simulink model "HWA1"  (R2017a)
settings: Solver=VariableStepAuto  StartTime=0.0  StopTime=10.0  RelTol=1e-3  EnableMultiTasking=on
values from neighbouring files (symbols this model uses):
  g = 9.81    [main.m]
  m = 0.4    [main.m]
settings Model: Creator=s160096  LastModifiedBy=Filip Davidovic
settings OptimizationCC: LifeSpan=inf
settings DebuggingCC: SFUnexpectedBacktrackingDiag=warning  SFNoUnconditionalDefaultTransitionDiag=warning  SFExecutionAtInitializationDiag=none
settings GRTTargetCC: TargetLangStandard=C89/C90 (ANSI)  GeneratePreprocessorConditionals=Disable all
settings ConfigComp: CovMetricSettings=dw  CovHtmlReporting=on  CovSaveCumulativeToWorkspaceVar=on  CovSaveSingleToWorkspaceVar=on  CovExternalEMLEnable=off

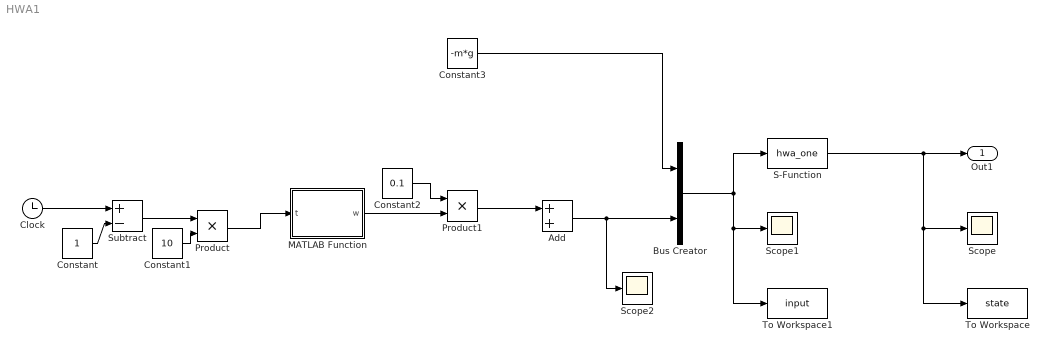
== system HWA1 ==
  Add : Sum
  Bus Creator : BusCreator  Inputs=2
  Clock : Clock
  Constant : Constant
  Constant1 : Constant  Value=10
  Constant2 : Constant  Value=0.1
  Constant3 : Constant  Value=-m*g
  MATLAB Function : MATLAB Function  TreatAsAtomicUnit=on
  Product : Product
  Product1 : Product
  S-Function : S-Function  FunctionName=hwa_one  Parameters=x0,g, m, ix, iy, iz  SFunctionModules=constants  SFunctionDeploymentMode=off  EnableBusSupport=off
  Scope : Scope
  Scope1 : Scope
  Scope2 : Scope
  Subtract : Sum  Inputs=+-
  To Workspace : ToWorkspace  VariableName=state  SaveFormat=Timeseries  SampleTime=-1
  To Workspace1 : ToWorkspace  VariableName=input  SaveFormat=Timeseries  SampleTime=-1
  Out1 : Outport
  wires:
  S-Function/1 -> To Workspace/1, Scope/1, Out1/1
  Bus Creator/1 -> To Workspace1/1, Scope1/1, S-Function/1
  MATLAB Function/1(w) -> Product1/2
  Clock/1 -> Subtract/1
  Constant/1 -> Subtract/2
  Subtract/1 -> Product/1
  Constant1/1 -> Product/2
  Product/1 -> MATLAB Function/1(t)
  Product1/1 -> Add/1
  Constant2/1 -> Product1/1
  Add/1 -> Scope2/1, Bus Creator/2
  Constant3/1 -> Bus Creator/1

== matlab function HWA1/MATLAB Function ==
  data: t input; w output
function w = wheaviside(t)
w = h(t)-2*h(t-1)+h(t-2);
